simulink model "SF033A_VehSigCdng"  (R2013b)
settings: Solver=FixedStepDiscrete  SolverMode=SingleTasking  StartTime=0.0  StopTime=1  FixedStep=.002  RelTol=1e-3
model workspace (MAT data in the model file):
  SLAMConfig_1_ATPP = [3707764736; 2; 1; 1; 1; 34]
values from neighbouring files (symbols this model uses):
  ARCHGLBPRM_2MILLISEC_SEC_F32 = DataDict.Constant    [SF033A_VehSigCdng_DataDict.m]
  ARCHGLBPRM_PIOVER180_ULS_F32 = DataDict.Constant    [SF033A_VehSigCdng_DataDict.m]
  AUNITCNVN_KPHPERSECPERMTRPERSECSQD_F32 = DataDict.Constant    [SF033A_VehSigCdng_DataDict.m]
  FLTINJ_VEHSIGCDNG_SERLCOMVEHLATA = DataDict.Constant    [SF033A_VehSigCdng_DataDict.m]
  FLTINJ_VEHSIGCDNG_SERLCOMVEHLGTA = DataDict.Constant    [SF033A_VehSigCdng_DataDict.m]
  FLTINJ_VEHSIGCDNG_SERLCOMVEHSPD = DataDict.Constant    [SF033A_VehSigCdng_DataDict.m]
  FLTINJ_VEHSIGCDNG_SERLCOMVEHYAWRATE = DataDict.Constant    [SF033A_VehSigCdng_DataDict.m]
  KPHCONVTOMTRPERSEC_MTRPERSECPERKPH_F32 = DataDict.Constant    [SF033A_VehSigCdng_DataDict.m]
  VehSigCdngDftLatA = DataDict.Calibration    [SF033A_VehSigCdng_DataDict.m]
  VehSigCdngDftLgtA = DataDict.Calibration    [SF033A_VehSigCdng_DataDict.m]
  VehSigCdngDftVehSpd = DataDict.Calibration    [SF033A_VehSigCdng_DataDict.m]
  VehSigCdngDftYawRate = DataDict.Calibration    [SF033A_VehSigCdng_DataDict.m]
  VehSigCdngLatADifThd = DataDict.Calibration    [SF033A_VehSigCdng_DataDict.m]
  VehSigCdngLatASlewRate = DataDict.Calibration    [SF033A_VehSigCdng_DataDict.m]
  VehSigCdngLtgADifThd = DataDict.Calibration    [SF033A_VehSigCdng_DataDict.m]
  VehSigCdngLtgASlewRate = DataDict.Calibration    [SF033A_VehSigCdng_DataDict.m]
  VehSigCdngVehSpdDifThd = DataDict.Calibration    [SF033A_VehSigCdng_DataDict.m]
  VehSigCdngVehSpdSlewRate = DataDict.Calibration    [SF033A_VehSigCdng_DataDict.m]
  VehSigCdngVehYawSlewRate = DataDict.Calibration    [SF033A_VehSigCdng_DataDict.m]
  VehSigCdngYawRateDifThd = DataDict.Calibration    [SF033A_VehSigCdng_DataDict.m]
  VEHSPDOVRDHWTQTHD_HWNWTMTR_F32 = DataDict.Constant    [SF033A_VehSigCdng_DataDict.m]
libraries: NxtrLim x9, CollectionOfReusableBlocks x6, Fil x4, simulink x1
(part 1 of 3)
settings Model: Creator=lzz0tm  LastModifiedBy=bzhf94
settings SolverCC: AutoInsertRateTranBlk=on  InsertRTBMode=Always
settings DataIOCC: LimitDataPoints=off  SaveFormat=Structure  ReturnWorkspaceOutputs=on
settings OptimizationCC: BlockReduction=off  InlineParams=on  ZeroExternalMemoryAtStartup=off  ZeroInternalMemoryAtStartup=off  OptimizeModelRefInitCode=on  LifeSpan=1
settings DebuggingCC: SignalInfNanChecking=error  SignalRangeChecking=warning  UnderspecifiedInitializationDetection=Simplified  SolverPrmCheckMsg=error  InheritedTsInSrcMsg=error  DiscreteInheritContinuousMsg=error  SingleTaskRateTransMsg=error  TasksWithSamePriorityMsg=error  SigSpecEnsureSampleTimeMsg=error  CheckMatrixSingularityMsg=error  ParameterUnderflowMsg=error  ParameterPrecisionLossMsg=error  ParameterTunabilityLossMsg=error  FixptConstUnderflowMsg=warning  FixptConstOverflowMsg=warning  VectorMatrixConversionMsg=error  SignalLabelMismatchMsg=error  UnconnectedInputMsg=error  UnconnectedOutputMsg=error  UnconnectedLineMsg=error  SFcnCompatibilityMsg=error  UniqueDataStoreMsg=warning  BusObjectLabelMismatch=error  RootOutportRequireBusObject=error  AssertControl=DisableAll  ModelReferenceIOMsg=error  ModelReferenceVersionMismatchMessage=warning  ModelReferenceIOMismatchMessage=error  ModelReferenceCSMismatchMessage=warning  ModelReferenceDataLoggingMessage=error  StateNameClashWarn=warning  StrictBusMsg=ErrorOnBusTreatedAsVector  NonBusSignalsTreatedAsBus=error  SFUnexpectedBacktrackingDiag=error  SFInvalidInputDataAccessInChartInitDiag=error  SFNoUnconditionalDefaultTransitionDiag=error  SFTransitionOutsideNaturalParentDiag=error  SFUnconditionalTransitionShadowingDiag=error  SFUndirectedBroadcastEventsDiag=error
settings ModelReferenceCC: ModelReferenceNumInstancesAllowed=Single
settings RTWCC: SystemTargetFile=autosar.tlc  GenCodeOnly=on  TemplateMakefile=ert_default_tmf  Description=AUTOSAR  GenerateReport=on  ProcessScript=autosar_make_rtw_hook  LaunchReport=on
settings CodeAppCC: GenerateComments=off  IgnoreCustomStorageClasses=off  CustomSymbolStrType=$N$R$M  CustomSymbolStrBlkIO=$N$M  SimulinkBlockComments=off
settings STFCustomTargetCC: ParMdlRefBuildCompliant=on  CompOptLevelCompliant=on  IncludeMdlTerminateFcn=off  CombineOutputUpdateFcns=on  SuppressErrorStatus=on  ERTFirstTimeCompliant=on  ERTCustomFileBanners=on  SupportNonFinite=off  SupportComplex=off  SupportContinuousTime=off  SupportNonInlinedSFcns=off  MATLABClassNameForMDSCustomization=Simulink.SoftwareTarget.ERTCustomization  AutosarCompliant=on  GRTInterface=off  SystemTargetFile=autosar.tlc
settings ERTTargetCC: CodeReplacementLibrary=ANSI_C  ConcurrentExecutionCompliant=off  IncludeMdlTerminateFcn=off  SuppressErrorStatus=on  SupportNonFinite=off  SupportComplex=off  ModelStepFunctionPrototypeControlCompliant=off  CPPClassGenCompliant=off  AutosarCompliant=on  InlinedParameterPlacement=NonHierarchical  ERTCustomFileTemplate=example_file_process.tlc  EnableUserReplacementTypes=on

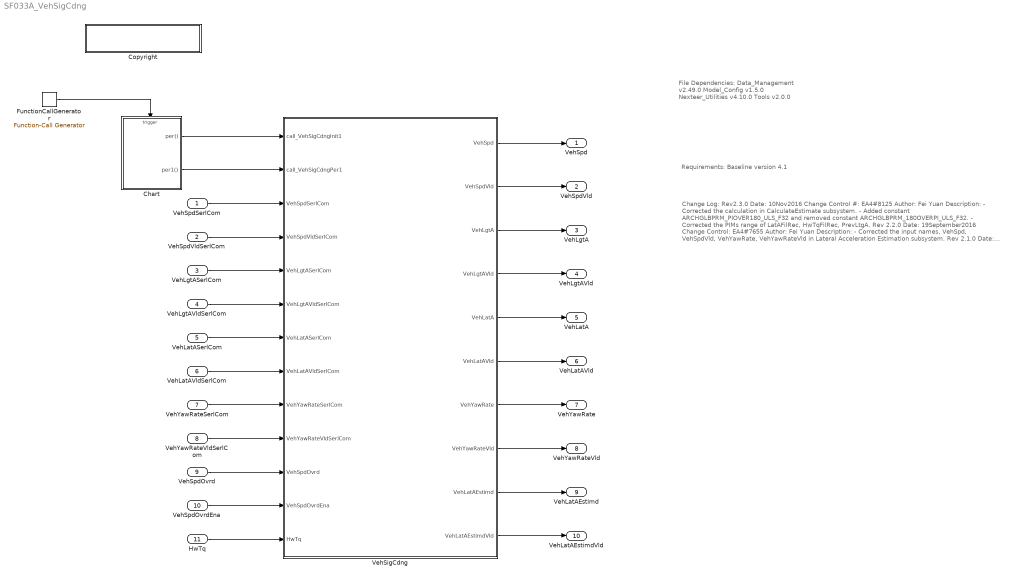
== system SF033A_VehSigCdng ==
  note: File Dependencies:
      |
      | Data_Management v2.49.0
      | Model_Config v1.5.0
      | Nexteer_Utilities v4.10.0
      | Tools v2.0.0
  note: Requirements: Baseline version 4.1
  note: Change Log:
      |
      | Rev2.3.0
      | Date: 10Nov2016
      | Change Control #: EA4#8125
      | Author: Fei Yuan
      | Description:
      | - Corrected the calculation in CalculateEstimate subsystem.
      | - Added constant ARCHGLBPRM_PIOVER180_ULS_F32 and removed constant
      |   ARCHGLBPRM_180OVERPI_ULS_F32.
      | - Corrected the PIMs range of LatAFilRec, HwTqFilRec, PrevLtgA.
      |
      |
      | Rev 2.2.0
      | Date: 19September2016
      | Change Control: EA4#7655
      | Author: Fei Yuan
      | Description:
      | - Corrected the input names, VehSpd, VehSpdVld, VehYawRate, VehYawRateVld in Lateral Acceleration
      | Estimation subsystem.
      |
      |
      | Rev 2.1.0
      | Date: 19August2016
      | Change Control: EA4#6834
      | Author P. Lefler
      | Description:
      | - Update the design so that VehLatAEstimd  is set to VehSpdDdngDftLatA when
      | VehLatAEstimdVld is FALSE and that VehLatAEstimd is calculated from VehSpd and VehYawRate instead of
      | the serial comm messages.
      |
      | - Correct the calculation of VehLatAEstimd. The constants applied to the VehYawRate and
      | VehSpd need to be interchanged.
      |
      |
      | Rev 2.0.0
      | Date: 24May2016
      | Change Control: EA4#3820, EA4#5691
      | Author: P. Lefler
      | Description:
      | EA4#3820 - The calculation and ouput of an estimated Lateral Accleration has been added with an output of validitiy
      | that is determined from the validity of the serial com input signals of Yaw Rate and Vehicle Speed.
      |
      | EA4#5691 - Added inputs and logic to provide override of Vehicle Speed for manufacturing.
      |
      | Rev: 1.1.0
      | Date :16-Oct-2015
      | Change Control #: EA4#2111
      | Author : Sudeep Shankar
      | Description:
      | - Data type of 'VehYawRateVldSerlCom'
      | changed to boolean.
      | - "Data type" of input and output ports changed
      |  to "Inherit: auto" ( Click on a port in the model and
      | select "Signal Attributes")
      |
      |
      | Rev: 1.0.0
      | Date: 26JUN2015
      | Change Control #: EA4#855
      | DRW: Wheatley
      | Description:
      | - Initial EA4 Release, based off
      | 	of EA3 4.0.0 release
  VehSpdSerlCom : Inport  PortDimensions=1
  VehSpdVldSerlCom : Inport  Port=2  PortDimensions=1
  VehLgtASerlCom : Inport  Port=3  PortDimensions=1
  VehLgtAVldSerlCom : Inport  Port=4  PortDimensions=1
  VehLatASerlCom : Inport  Port=5  PortDimensions=1
  VehLatAVldSerlCom : Inport  Port=6  PortDimensions=1
  VehYawRateSerlCom : Inport  Port=7  PortDimensions=1
  VehYawRateVldSerlCom : Inport  Port=8  PortDimensions=1
  VehSpdOvrd : Inport  Port=9  PortDimensions=1
  VehSpdOvrdEna : Inport  Port=10  PortDimensions=1
  HwTq : Inport  Port=11  PortDimensions=1
  Chart : Stateflow chart  TreatAsAtomicUnit=on
  Copyright : Subsystem  Description=|  mask(Copyright Information){none=on}
      | Copyright info block.                                               
      |                                                                     
      | Place copyright information at the top of every subsystem in design.
      mask prompts: none "No parameters"
      mask help: Place copyright information at the top of every subsystem in design.
      mask Display:
      | NxtrConf = 'Nexteer Confidential';
      | 
      | sys = bdroot; %handle for the current model ("system")
      | first = get_param(sys,'Created');
      | first = first(end-3:end);  %year is last four digits
      | 
      | last = get_param(sys,'LastModifiedDate');
      | if isempty(last)
      |     last = datestr(now,'yyyy');
      | else
      |     last = last(end-3:end);
      | end
      | 
      | if strcmp(first,last)
      |     fprintf('%s\nCopyright  %s Nexteer',NxtrConf,first);
      | else
      |     fprintf('%s\n%s%s-%s Nexteer',NxtrConf,char(169),first,last);
      | end
  FunctionCallGenerator : simulink/Ports & Subsystems/Function-Call Generator  sample_time=0.002  numberOfIterations=1
  VehSigCdng : Subsystem
  VehSpd : Outport  PortDimensions=1
  VehSpdVld : Outport  Port=2  PortDimensions=1
  VehLgtA : Outport  Port=3  PortDimensions=1
  VehLgtAVld : Outport  Port=4  PortDimensions=1
  VehLatA : Outport  Port=5  PortDimensions=1
  VehLatAVld : Outport  Port=6  PortDimensions=1
  VehYawRate : Outport  Port=7  PortDimensions=1
  VehYawRateVld : Outport  Port=8  PortDimensions=1
  VehLatAEstimd : Outport  Port=9
  VehLatAEstimdVld : Outport  Port=10
  wires:
  VehLgtASerlCom/1 -> VehSigCdng/5(VehLgtASerlCom)
  VehLgtAVldSerlCom/1 -> VehSigCdng/6(VehLgtAVldSerlCom)
  VehLatASerlCom/1 -> VehSigCdng/7(VehLatASerlCom)
  VehLatAVldSerlCom/1 -> VehSigCdng/8(VehLatAVldSerlCom)
  VehYawRateSerlCom/1 -> VehSigCdng/9(VehYawRateSerlCom)
  VehYawRateVldSerlCom/1 -> VehSigCdng/10(VehYawRateVldSerlCom)
  VehSigCdng/1(VehSpd) -> VehSpd/1
  VehSigCdng/2(VehSpdVld) -> VehSpdVld/1
  VehSigCdng/3(VehLgtA) -> VehLgtA/1
  VehSigCdng/4(VehLgtAVld) -> VehLgtAVld/1
  VehSigCdng/5(VehLatA) -> VehLatA/1
  VehSigCdng/6(VehLatAVld) -> VehLatAVld/1
  VehSigCdng/7(VehYawRate) -> VehYawRate/1
  VehSigCdng/8(VehYawRateVld) -> VehYawRateVld/1
  FunctionCallGenerator/1 -> Chart/Trigger
  Chart/1(per()) -> VehSigCdng/1(call_VehSigCdngInit1)
  Chart/2(per1()) -> VehSigCdng/2(call_VehSigCdngPer1)
  VehSigCdng/9(VehLatAEstimd) -> VehLatAEstimd/1
  VehSigCdng/10(VehLatAEstimdVld) -> VehLatAEstimdVld/1
  VehSpdVldSerlCom/1 -> VehSigCdng/4(VehSpdVldSerlCom)
  VehSpdSerlCom/1 -> VehSigCdng/3(VehSpdSerlCom)
  VehSpdOvrdEna/1 -> VehSigCdng/12(VehSpdOvrdEna)
  HwTq/1 -> VehSigCdng/13(HwTq)
  VehSpdOvrd/1 -> VehSigCdng/11(VehSpdOvrd)

== system SF033A_VehSigCdng/Copyright ==

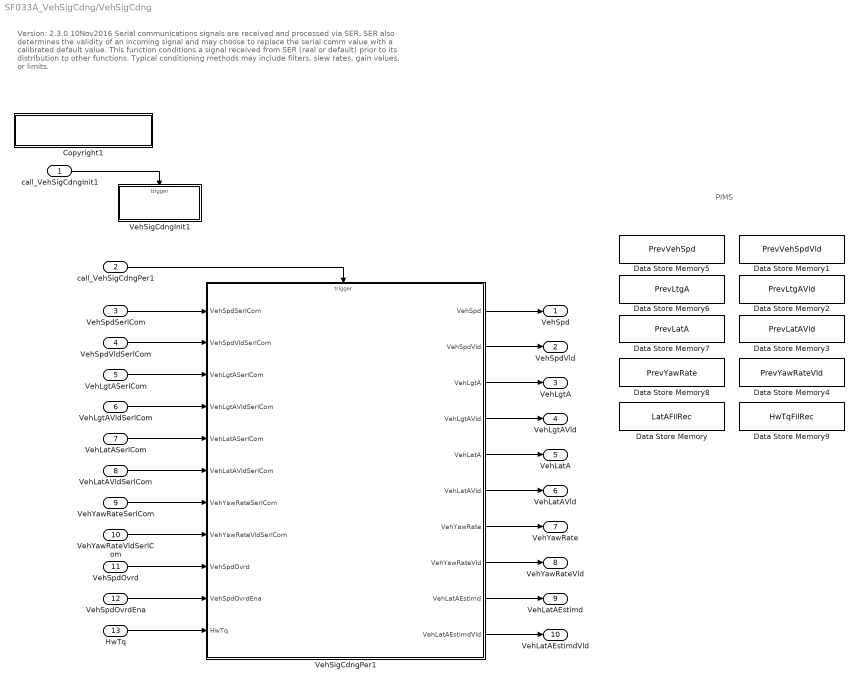
== system SF033A_VehSigCdng/VehSigCdng ==
  note: PIMS
  note: Version:  2.3.0				10Nov2016
      |
      | Serial communications signals are received and processed via SER.  SER also determines the validity of an incoming signal and may choose to replace the serial comm value with a calibrated default value.
      | This function conditions a signal received from SER (real or default) prior to its distribution to other functions.  Typical conditioning methods may include filters, slew rates, gain values, or limits.
  call_VehSigCdngInit1 : Inport
  call_VehSigCdngPer1 : Inport  Port=2
  VehSpdSerlCom : Inport  RequirementInfo="{'linktype_rmi_doors' '00012fc2 (/E-STEER Core/SubSystem Specifications/Application Functions - EA4/SF033A Vehicle Signal Conditioning)' '#SF033A_9' 'true' 'REQ:  SF033A_9' '' } %GIDa_54d4a7a3_9b19_443d_8fc5_eee67838605b"  Port=3  PortDimensions=1
  VehSpdVldSerlCom : Inport  RequirementInfo="{'linktype_rmi_doors' '00012fc2 (/E-STEER Core/SubSystem Specifications/Application Functions - EA4/SF033A Vehicle Signal Conditioning)' '#SF033A_48' 'true' 'REQ:  SF033A_48' '' } %GIDa_072279f1_3b2c_44d1_aaac_d278ed9b7397"  Port=4  PortDimensions=1
  VehLgtASerlCom : Inport  RequirementInfo="{'linktype_rmi_doors' '00012fc2 (/E-STEER Core/SubSystem Specifications/Application Functions - EA4/SF033A Vehicle Signal Conditioning)' '#SF033A_49' 'true' 'REQ:  SF033A_49' '' } %GIDa_26c8abc2_7194_48ce_90af_9aea8ac14bea"  Port=5  PortDimensions=1
  VehLgtAVldSerlCom : Inport  RequirementInfo="{'linktype_rmi_doors' '00012fc2 (/E-STEER Core/SubSystem Specifications/Application Functions - EA4/SF033A Vehicle Signal Conditioning)' '#SF033A_50' 'true' 'REQ:  SF033A_50' '' } %GIDa_37f55aeb_95e9_4e82_a468_aabd9ebeee97"  Port=6  PortDimensions=1
  VehLatASerlCom : Inport  RequirementInfo="{'linktype_rmi_doors' '00012fc2 (/E-STEER Core/SubSystem Specifications/Application Functions - EA4/SF033A Vehicle Signal Conditioning)' '#SF033A_51' 'true' 'REQ:  SF033A_51' '' } %GIDa_d8fc8d11_e171_48fe_b9fc_d65fe4604617"  Port=7  PortDimensions=1
  VehLatAVldSerlCom : Inport  RequirementInfo="{'linktype_rmi_doors' '00012fc2 (/E-STEER Core/SubSystem Specifications/Application Functions - EA4/SF033A Vehicle Signal Conditioning)' '#SF033A_52' 'true' 'REQ:  SF033A_52' '' } %GIDa_d1cab1a5_fbf5_438a_a129_ecd49d66000b"  Port=8  PortDimensions=1
  VehYawRateSerlCom : Inport  RequirementInfo="{'linktype_rmi_doors' '00012fc2 (/E-STEER Core/SubSystem Specifications/Application Functions - EA4/SF033A Vehicle Signal Conditioning)' '#SF033A_53' 'true' 'REQ:  SF033A_53' '' } %GIDa_e3d4cf11_eb0a_4628_8932_e44618244c7f"  Port=9  PortDimensions=1
  VehYawRateVldSerlCom : Inport  RequirementInfo="{'linktype_rmi_doors' '00012fc2 (/E-STEER Core/SubSystem Specifications/Application Functions - EA4/SF033A Vehicle Signal Conditioning)' '#SF033A_54' 'true' 'REQ:  SF033A_54' '' } %GIDa_0d1894a8_7423_4afc_9a9d_b2e7187f4361"  Port=10  PortDimensions=1
  VehSpdOvrd : Inport  RequirementInfo="{'linktype_rmi_doors' '00012fc2 (/E-STEER Core/SubSystem Specifications/Application Functions - EA4/SF033A Vehicle Signal Conditioning)' '#SF033A_55' 'true' 'REQ:  SF033A_55' '' } %GIDa_6a43a7d4_88db_4c6f_8f53_b974adffb088"  Port=11  PortDimensions=1
  VehSpdOvrdEna : Inport  RequirementInfo="{'linktype_rmi_doors' '00012fc2 (/E-STEER Core/SubSystem Specifications/Application Functions - EA4/SF033A Vehicle Signal Conditioning)' '#SF033A_56' 'true' 'REQ:  SF033A_56' '' } %GIDa_18bae755_d713_41e5_97b7_5a248150ee5f"  Port=12  PortDimensions=1
  HwTq : Inport  RequirementInfo="{'linktype_rmi_doors' '00012fc2 (/E-STEER Core/SubSystem Specifications/Application Functions - EA4/SF033A Vehicle Signal Conditioning)' '#SF033A_57' 'true' 'REQ:  SF033A_57' '' } %GIDa_76451758_dfda_400b_b021_5024d294a7ba"  Port=13  PortDimensions=1
  Copyright1 : Subsystem  Description=|  mask(Copyright Information){none=on}
      | Copyright info block.                                               
      |                                                                     
      | Place copyright information at the top of every subsystem in design.
      mask prompts: none "No parameters"
      mask help: Place copyright information at the top of every subsystem in design.
      mask Display:
      | NxtrConf = 'Nexteer Confidential';
      | 
      | sys = bdroot; %handle for the current model ("system")
      | first = get_param(sys,'Created');
      | first = first(end-3:end);  %year is last four digits
      | 
      | last = get_param(sys,'LastModifiedDate');
      | if isempty(last)
      |     last = datestr(now,'yyyy');
      | else
      |     last = last(end-3:end);
      | end
      | 
      | if strcmp(first,last)
      |     fprintf('%s\nCopyright  %s Nexteer',NxtrConf,first);
      | else
      |     fprintf('%s\n%s%s-%s Nexteer',NxtrConf,char(169),first,last);
      | end
  Data Store Memory : DataStoreMemory  RequirementInfo="{'linktype_rmi_doors' '00012fc2 (/E-STEER Core/SubSystem Specifications/Application Functions - EA4/SF033A Vehicle Signal Conditioning)' '#SF033A_95' 'true' 'REQ:  SF033A_95' '' } %GIDa_0c5846ab_92bd_4d29_8a45_462a927c3a81"  DataStoreName=LatAFilRec  InitialValue=struct('FilSt',single(0),'FilGain',single(0))  OutDataTypeStr=Bus: FilLpRec1  StateMustResolveToSignalObject=on
  Data Store Memory1 : DataStoreMemory  DataStoreName=PrevVehSpdVld  StateMustResolveToSignalObject=on
  Data Store Memory2 : DataStoreMemory  DataStoreName=PrevLtgAVld  StateMustResolveToSignalObject=on
  Data Store Memory3 : DataStoreMemory  DataStoreName=PrevLatAVld  StateMustResolveToSignalObject=on
  Data Store Memory4 : DataStoreMemory  DataStoreName=PrevYawRateVld  StateMustResolveToSignalObject=on
  Data Store Memory5 : DataStoreMemory  DataStoreName=PrevVehSpd  StateMustResolveToSignalObject=on
  Data Store Memory6 : DataStoreMemory  DataStoreName=PrevLtgA  StateMustResolveToSignalObject=on
  Data Store Memory7 : DataStoreMemory  DataStoreName=PrevLatA  StateMustResolveToSignalObject=on
  Data Store Memory8 : DataStoreMemory  DataStoreName=PrevYawRate  StateMustResolveToSignalObject=on
  Data Store Memory9 : DataStoreMemory  RequirementInfo="{'linktype_rmi_doors' '00012fc2 (/E-STEER Core/SubSystem Specifications/Application Functions - EA4/SF033A Vehicle Signal Conditioning)' '#SF033A_70' 'true' 'REQ:  SF033A_70' '' ; 'linktype_rmi_doors' '00012fc2 (/E-STEER Core/SubSystem Specifications/Application Functions - EA4/SF033A Vehicle Signal Conditioning)' '#SF033A_106' 'true' 'REQ:  SF033A_106' '' } %GIDa_2e2802be_6404_4db6_874c_aabd103a4acc"  DataStoreName=HwTqFilRec  InitialValue=[]  StateMustResolveToSignalObject=on
  VehSigCdngInit1 : Subsystem  TreatAsAtomicUnit=on
  VehSigCdngPer1 : Subsystem
  VehSpd : Outport  RequirementInfo="{'linktype_rmi_doors' '00012fc2 (/E-STEER Core/SubSystem Specifications/Application Functions - EA4/SF033A Vehicle Signal Conditioning)' '#SF033A_11' 'true' 'REQ:  SF033A_11' '' } %GIDa_233b96dc_1a76_410d_9511_57228fcb2a2c"  PortDimensions=1
  VehSpdVld : Outport  RequirementInfo="{'linktype_rmi_doors' '00012fc2 (/E-STEER Core/SubSystem Specifications/Application Functions - EA4/SF033A Vehicle Signal Conditioning)' '#SF033A_58' 'true' 'REQ:  SF033A_58' '' } %GIDa_ac8eeb31_52c9_4a8f_b3bc_984b37742cf2"  Port=2  PortDimensions=1
  VehLgtA : Outport  RequirementInfo="{'linktype_rmi_doors' '00012fc2 (/E-STEER Core/SubSystem Specifications/Application Functions - EA4/SF033A Vehicle Signal Conditioning)' '#SF033A_59' 'true' 'REQ:  SF033A_59' '' } %GIDa_690e0b41_3963_43a6_9a31_eb7586529f9d"  Port=3  PortDimensions=1
  VehLgtAVld : Outport  RequirementInfo="{'linktype_rmi_doors' '00012fc2 (/E-STEER Core/SubSystem Specifications/Application Functions - EA4/SF033A Vehicle Signal Conditioning)' '#SF033A_61' 'true' 'REQ:  SF033A_61' '' } %GIDa_d05753c6_a2a8_4d16_8807_9f672ca9e552"  Port=4  PortDimensions=1
  VehLatA : Outport  RequirementInfo="{'linktype_rmi_doors' '00012fc2 (/E-STEER Core/SubSystem Specifications/Application Functions - EA4/SF033A Vehicle Signal Conditioning)' '#SF033A_62' 'true' 'REQ:  SF033A_62' '' } %GIDa_87d4c65b_0136_48cb_a577_93593ee03691"  Port=5  PortDimensions=1
  VehLatAVld : Outport  RequirementInfo="{'linktype_rmi_doors' '00012fc2 (/E-STEER Core/SubSystem Specifications/Application Functions - EA4/SF033A Vehicle Signal Conditioning)' '#SF033A_65' 'true' 'REQ:  SF033A_65' '' } %GIDa_16cef6e8_4176_4268_935b_383d23a79d5c"  Port=6  PortDimensions=1
  VehYawRate : Outport  RequirementInfo="{'linktype_rmi_doors' '00012fc2 (/E-STEER Core/SubSystem Specifications/Application Functions - EA4/SF033A Vehicle Signal Conditioning)' '#SF033A_63' 'true' 'REQ:  SF033A_63' '' } %GIDa_5922fcb3_f223_4d4a_a6ba_bb2ffcc33926"  Port=7  PortDimensions=1
  VehYawRateVld : Outport  RequirementInfo="{'linktype_rmi_doors' '00012fc2 (/E-STEER Core/SubSystem Specifications/Application Functions - EA4/SF033A Vehicle Signal Conditioning)' '#SF033A_64' 'true' 'REQ:  SF033A_64' '' } %GIDa_ede16489_acab_444a_8f38_7e62a6621c77"  Port=8  PortDimensions=1
  VehLatAEstimd : Outport  RequirementInfo="{'linktype_rmi_doors' '00012fc2 (/E-STEER Core/SubSystem Specifications/Application Functions - EA4/SF033A Vehicle Signal Conditioning)' '#SF033A_60' 'true' 'REQ:  SF033A_60' '' } %GIDa_bd1c9d75_d3fa_4d5a_9ec3_8a13a125d70d"  Port=9
  VehLatAEstimdVld : Outport  RequirementInfo="{'linktype_rmi_doors' '00012fc2 (/E-STEER Core/SubSystem Specifications/Application Functions - EA4/SF033A Vehicle Signal Conditioning)' '#SF033A_66' 'true' 'REQ:  SF033A_66' '' } %GIDa_e77b9470_d33a_498a_a2de_20107a9a1a32"  Port=10
  wires:
  VehLgtASerlCom/1 -> VehSigCdngPer1/3(VehLgtASerlCom)
  VehSpdSerlCom/1 -> VehSigCdngPer1/1(VehSpdSerlCom)
  call_VehSigCdngPer1/1 -> VehSigCdngPer1/Trigger
  VehSpdVldSerlCom/1 -> VehSigCdngPer1/2(VehSpdVldSerlCom)
  VehLatASerlCom/1 -> VehSigCdngPer1/5(VehLatASerlCom)
  call_VehSigCdngInit1/1 -> VehSigCdngInit1/Trigger
  VehLgtAVldSerlCom/1 -> VehSigCdngPer1/4(VehLgtAVldSerlCom)
  VehLatAVldSerlCom/1 -> VehSigCdngPer1/6(VehLatAVldSerlCom)
  VehYawRateSerlCom/1 -> VehSigCdngPer1/7(VehYawRateSerlCom)
  VehYawRateVldSerlCom/1 -> VehSigCdngPer1/8(VehYawRateVldSerlCom)
  VehSigCdngPer1/1(VehSpd) -> VehSpd/1
  VehSigCdngPer1/2(VehSpdVld) -> VehSpdVld/1
  VehSigCdngPer1/3(VehLgtA) -> VehLgtA/1
  VehSigCdngPer1/5(VehLatA) -> VehLatA/1
  VehSigCdngPer1/4(VehLgtAVld) -> VehLgtAVld/1
  VehSigCdngPer1/6(VehLatAVld) -> VehLatAVld/1
  VehSigCdngPer1/7(VehYawRate) -> VehYawRate/1
  VehSigCdngPer1/8(VehYawRateVld) -> VehYawRateVld/1
  VehSigCdngPer1/9(VehLatAEstimd) -> VehLatAEstimd/1
  VehSigCdngPer1/10(VehLatAEstimdVld) -> VehLatAEstimdVld/1
  VehSpdOvrd/1 -> VehSigCdngPer1/9(VehSpdOvrd)
  VehSpdOvrdEna/1 -> VehSigCdngPer1/10(VehSpdOvrdEna)
  HwTq/1 -> VehSigCdngPer1/11(HwTq)

== system SF033A_VehSigCdng/VehSigCdng/Copyright1 ==

== system SF033A_VehSigCdng/VehSigCdng/VehSigCdngInit1 ==
  function : TriggerPort  TriggerType=function-call
  CopyRight2 : Subsystem  Description=|  mask(Copyright Information){none=on}
      | Copyright info block.                                               
      |                                                                     
      | Place copyright information at the top of every subsystem in design.
      mask prompts: none "No parameters"
      mask help: Place copyright information at the top of every subsystem in design.
      mask Display:
      | NxtrConf = 'Nexteer Confidential';
      | 
      | sys = bdroot; %handle for the current model ("system")
      | first = get_param(sys,'Created');
      | first = first(end-3:end);  %year is last four digits
      | 
      | last = get_param(sys,'LastModifiedDate');
      | if isempty(last)
      |     last = datestr(now,'yyyy');
      | else
      |     last = last(end-3:end);
      | end
      | 
      | if strcmp(first,last)
      |     fprintf('%s -- Copyright %s Nexteer',NxtrConf,first)
      | else
      |     fprintf('%s -- %s%s- %s Nexteer',NxtrConf,char(169),first,last)
      | end
  FilLpInit : Fil/FilLpInit  RequirementInfo="{'linktype_rmi_doors' '00012fc2 (/E-STEER Core/SubSystem Specifications/Application Functions - EA4/SF033A Vehicle Signal Conditioning)' '#SF033A_95' 'true' 'REQ:  SF033A_95' '' } %GIDa_7accb8cc_27e6_4227_a4fe_4cab8debe218"  Ic=0  Ts=ARCHGLBPRM_2MILLISEC_SEC_F32  Freq=VehSigCdngLatAFilFrq  StVar=LatAFilRec
  FilLpInit1 : Fil/FilLpInit  RequirementInfo="{'linktype_rmi_doors' '00012fc2 (/E-STEER Core/SubSystem Specifications/Application Functions - EA4/SF033A Vehicle Signal Conditioning)' '#SF033A_70' 'true' 'REQ:  SF033A_70' '' ; 'linktype_rmi_doors' '00012fc2 (/E-STEER Core/SubSystem Specifications/Application Functions - EA4/SF033A Vehicle Signal Conditioning)' '#SF033A_106' 'true' 'REQ:  SF033A_106' '' } %GIDa_a1695ab3_73dc_4f0d_88aa_6746bdcfefc1"  Ic=0  Ts=ARCHGLBPRM_2MILLISEC_SEC_F32  Freq=single(0.1)  StVar=HwTqFilRec

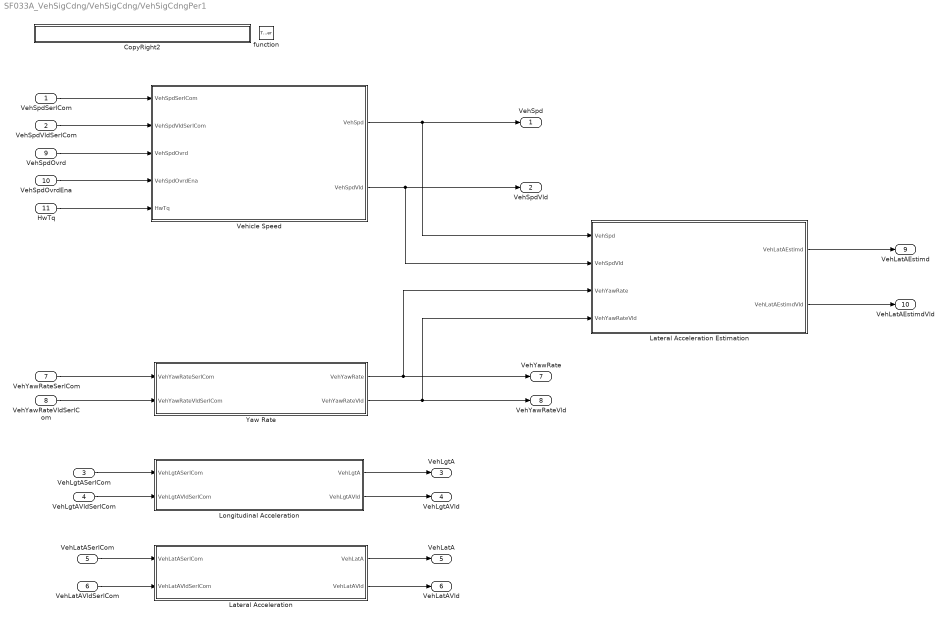
== system SF033A_VehSigCdng/VehSigCdng/VehSigCdngPer1 ==
  VehSpdSerlCom : Inport  PortDimensions=1
  VehSpdVldSerlCom : Inport  Port=2  PortDimensions=1
  VehLgtASerlCom : Inport  Port=3  PortDimensions=1
  VehLgtAVldSerlCom : Inport  Port=4  PortDimensions=1
  VehLatASerlCom : Inport  Port=5  PortDimensions=1
  VehLatAVldSerlCom : Inport  Port=6  PortDimensions=1
  VehYawRateSerlCom : Inport  Port=7  PortDimensions=1
  VehYawRateVldSerlCom : Inport  Port=8  PortDimensions=1
  VehSpdOvrd : Inport  Port=9  PortDimensions=1
  VehSpdOvrdEna : Inport  Port=10  PortDimensions=1
  HwTq : Inport  Port=11  PortDimensions=1
  function : TriggerPort  TriggerType=function-call  PortDimensions=1
  CopyRight2 : Subsystem  Description=|  mask(Copyright Information){none=on}
      | Copyright info block.                                               
      |                                                                     
      | Place copyright information at the top of every subsystem in design.
      mask prompts: none "No parameters"
      mask help: Place copyright information at the top of every subsystem in design.
      mask Display:
      | NxtrConf = 'Nexteer Confidential';
      | 
      | sys = bdroot; %handle for the current model ("system")
      | first = get_param(sys,'Created');
      | first = first(end-3:end);  %year is last four digits
      | 
      | last = get_param(sys,'LastModifiedDate');
      | if isempty(last)
      |     last = datestr(now,'yyyy');
      | else
      |     last = last(end-3:end);
      | end
      | 
      | if strcmp(first,last)
      |     fprintf('%s -- Copyright %s Nexteer',NxtrConf,first)
      | else
      |     fprintf('%s -- %s%s- %s Nexteer',NxtrConf,char(169),first,last)
      | end
  Lateral Acceleration : Subsystem
  Lateral Acceleration Estimation : Subsystem
  Longitudinal Acceleration : Subsystem
  Vehicle Speed : Subsystem
  "Yaw Rate " : Subsystem
  VehSpd : Outport  PortDimensions=1
  VehSpdVld : Outport  Port=2  PortDimensions=1
  VehLgtA : Outport  Port=3  PortDimensions=1
  VehLgtAVld : Outport  Port=4  PortDimensions=1
  VehLatA : Outport  Port=5  PortDimensions=1
  VehLatAVld : Outport  Port=6  PortDimensions=1
  VehYawRate : Outport  Port=7  PortDimensions=1
  VehYawRateVld : Outport  Port=8  PortDimensions=1
  VehLatAEstimd : Outport  Port=9
  VehLatAEstimdVld : Outport  Port=10
  wires:
  Vehicle Speed/1(VehSpd) -> VehSpd/1, Lateral Acceleration Estimation/1(VehSpd)
  Vehicle Speed/2(VehSpdVld) -> VehSpdVld/1, Lateral Acceleration Estimation/2(VehSpdVld)
  VehLgtASerlCom/1 -> Longitudinal Acceleration/1(VehLgtASerlCom)
  VehLgtAVldSerlCom/1 -> Longitudinal Acceleration/2(VehLgtAVldSerlCom)
  Longitudinal Acceleration/1(VehLgtA) -> VehLgtA/1
  Longitudinal Acceleration/2(VehLgtAVld) -> VehLgtAVld/1
  VehLatASerlCom/1 -> Lateral Acceleration/1(VehLatASerlCom)
  VehLatAVldSerlCom/1 -> Lateral Acceleration/2(VehLatAVldSerlCom)
  Lateral Acceleration/1(VehLatA) -> VehLatA/1
  Lateral Acceleration/2(VehLatAVld) -> VehLatAVld/1
  "Yaw Rate "/1(VehYawRate) -> Lateral Acceleration Estimation/3(VehYawRate), VehYawRate/1
  "Yaw Rate "/2(VehYawRateVld) -> Lateral Acceleration Estimation/4(VehYawRateVld), VehYawRateVld/1
  Lateral Acceleration Estimation/2(VehLatAEstimdVld) -> VehLatAEstimdVld/1
  Lateral Acceleration Estimation/1(VehLatAEstimd) -> VehLatAEstimd/1
  VehSpdSerlCom/1 -> Vehicle Speed/1(VehSpdSerlCom)
  VehYawRateSerlCom/1 -> "Yaw Rate "/1(VehYawRateSerlCom)
  VehSpdVldSerlCom/1 -> Vehicle Speed/2(VehSpdVldSerlCom)
  VehYawRateVldSerlCom/1 -> "Yaw Rate "/2(VehYawRateVldSerlCom)
  VehSpdOvrd/1 -> Vehicle Speed/3(VehSpdOvrd)
  VehSpdOvrdEna/1 -> Vehicle Speed/4(VehSpdOvrdEna)
  HwTq/1 -> Vehicle Speed/5(HwTq)

== system SF033A_VehSigCdng/VehSigCdng/VehSigCdngInit1/CopyRight2 ==

== system SF033A_VehSigCdng/VehSigCdng/VehSigCdngPer1/CopyRight2 ==

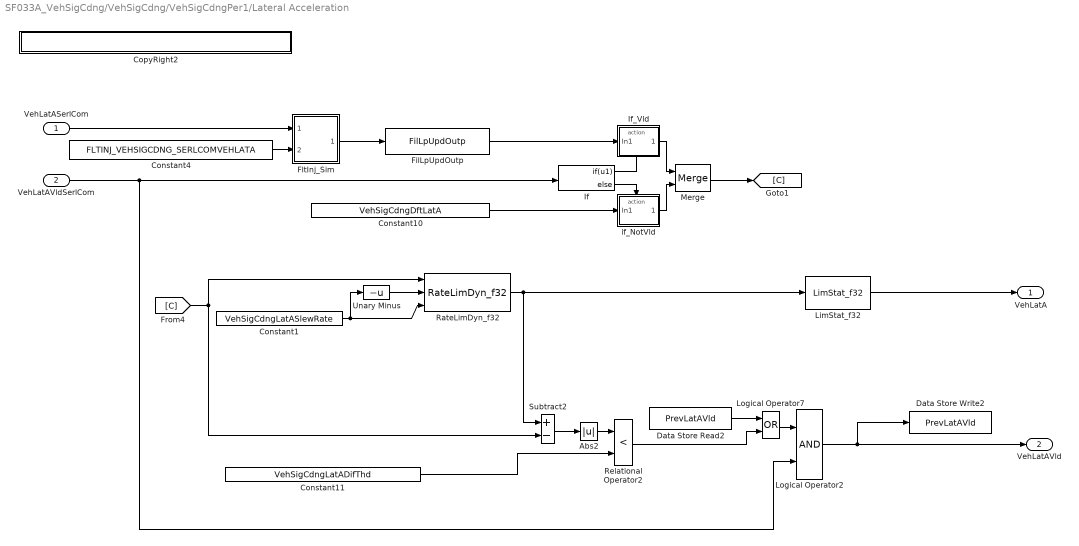
== system SF033A_VehSigCdng/VehSigCdng/VehSigCdngPer1/Lateral Acceleration ==
  VehLatASerlCom : Inport  RequirementInfo="{'linktype_rmi_doors' '00012fc2 (/E-STEER Core/SubSystem Specifications/Application Functions - EA4/SF033A Vehicle Signal Conditioning)' '#SF033A_95' 'true' 'REQ:  SF033A_95' '' ; 'linktype_rmi_doors' '00012fc2 (/E-STEER Core/SubSystem Specifications/Application Functions - EA4/SF033A Vehicle Signal Conditioning)' '#SF033A_96' 'true' 'REQ:  SF033A_96' '' } %GIDa_c753c921_7e04_496c_95fa_487e63ca1125"  PortDimensions=1
  VehLatAVldSerlCom : Inport  RequirementInfo="{'linktype_rmi_doors' '00012fc2 (/E-STEER Core/SubSystem Specifications/Application Functions - EA4/SF033A Vehicle Signal Conditioning)' '#SF033A_95' 'true' 'REQ:  SF033A_95' '' ; 'linktype_rmi_doors' '00012fc2 (/E-STEER Core/SubSystem Specifications/Application Functions - EA4/SF033A Vehicle Signal Conditioning)' '#SF033A_96' 'true' 'REQ:  SF033A_96' '' } %GIDa_b07f8488_028f_4994_885b_452029bb587c"  Port=2  PortDimensions=1
  Abs2 : Abs  RequirementInfo="{'linktype_rmi_doors' '00012fc2 (/E-STEER Core/SubSystem Specifications/Application Functions - EA4/SF033A Vehicle Signal Conditioning)' '#SF033A_94' 'true' 'REQ:  SF033A_94' '' } %GIDa_5a62b5de_cc32_48b8_924f_7873d67ebb50"
  Constant1 : Constant  RequirementInfo="{'linktype_rmi_doors' '00012fc2 (/E-STEER Core/SubSystem Specifications/Application Functions - EA4/SF033A Vehicle Signal Conditioning)' '#SF033A_92' 'true' 'REQ:  SF033A_92' '' } %GIDa_eb3c9be8_1e78_47b8_835b_b4d0d1ae4ea5"  Value=VehSigCdngLatASlewRate
  Constant10 : Constant  RequirementInfo="{'linktype_rmi_doors' '00012fc2 (/E-STEER Core/SubSystem Specifications/Application Functions - EA4/SF033A Vehicle Signal Conditioning)' '#SF033A_96' 'true' 'REQ:  SF033A_96' '' } %GIDa_91ae6bfc_aa5f_43f0_9820_b24db602beb2"  Value=VehSigCdngDftLatA
  Constant11 : Constant  RequirementInfo="{'linktype_rmi_doors' '00012fc2 (/E-STEER Core/SubSystem Specifications/Application Functions - EA4/SF033A Vehicle Signal Conditioning)' '#SF033A_94' 'true' 'REQ:  SF033A_94' '' } %GIDa_a0d1b654_bbde_4064_8b63_104446a06a98"  Value=VehSigCdngLatADifThd
  Constant4 : Constant  RequirementInfo="{'linktype_rmi_doors' '00012fc2 (/E-STEER Core/SubSystem Specifications/Application Functions - EA4/SF033A Vehicle Signal Conditioning)' '#SF033A_109' 'true' 'REQ:  SF033A_109' '' } %GIDa_1542dcc9_2bda_4046_a838_588fdf05564c"  Value=FLTINJ_VEHSIGCDNG_SERLCOMVEHLATA
  CopyRight2 : Subsystem  Description=|  mask(Copyright Information){none=on}
      | Copyright info block.                                               
      |                                                                     
      | Place copyright information at the top of every subsystem in design.
      mask prompts: none "No parameters"
      mask help: Place copyright information at the top of every subsystem in design.
      mask Display:
      | NxtrConf = 'Nexteer Confidential';
      | 
      | sys = bdroot; %handle for the current model ("system")
      | first = get_param(sys,'Created');
      | first = first(end-3:end);  %year is last four digits
      | 
      | last = get_param(sys,'LastModifiedDate');
      | if isempty(last)
      |     last = datestr(now,'yyyy');
      | else
      |     last = last(end-3:end);
      | end
      | 
      | if strcmp(first,last)
      |     fprintf('%s -- Copyright %s Nexteer',NxtrConf,first)
      | else
      |     fprintf('%s -- %s%s- %s Nexteer',NxtrConf,char(169),first,last)
      | end
  Data Store Read2 : DataStoreRead  DataStoreName=PrevLatAVld
  Data Store Write2 : DataStoreWrite  DataStoreName=PrevLatAVld
  FilLpUpdOutp : Fil/FilLpUpdOutp  RequirementInfo="{'linktype_rmi_doors' '00012fc2 (/E-STEER Core/SubSystem Specifications/Application Functions - EA4/SF033A Vehicle Signal Conditioning)' '#SF033A_95' 'true' 'REQ:  SF033A_95' '' } %GIDa_7953da50_dcec_437e_8f3a_a91fadd74616"  StVar=LatAFilRec
      settings: AttributesFormatString=StVar: %<StVar>
  FltInj_Sim : Subsystem  RequirementInfo="{'linktype_rmi_doors' '00012fc2 (/E-STEER Core/SubSystem Specifications/Application Functions - EA4/SF033A Vehicle Signal Conditioning)' '#SF033A_109' 'true' 'REQ:  SF033A_109' '' } %GIDa_932a3e69_52ef_4461_8f18_f05710d5a38c"  TreatAsAtomicUnit=on  VariantControl=FltInj_sim
  If : If  RequirementInfo="{'linktype_rmi_doors' '00012fc2 (/E-STEER Core/SubSystem Specifications/Application Functions - EA4/SF033A Vehicle Signal Conditioning)' '#SF033A_95' 'true' 'REQ:  SF033A_95' '' } %GIDa_c0a6e30e_f7f2_4ae2_8bd5_78b2454898f8"  IfExpression=u1
  If_Vld : Subsystem  RequirementInfo="{'linktype_rmi_doors' '00012fc2 (/E-STEER Core/SubSystem Specifications/Application Functions - EA4/SF033A Vehicle Signal Conditioning)' '#SF033A_95' 'true' 'REQ:  SF033A_95' '' } %GIDa_1a18b11a_c2c8_4315_9c86_e615b348a758"  TreatAsAtomicUnit=on
  LimStat_f32 : NxtrLim/LimStat_f32  RequirementInfo="{'linktype_rmi_doors' '00012fc2 (/E-STEER Core/SubSystem Specifications/Application Functions - EA4/SF033A Vehicle Signal Conditioning)' '#SF033A_68' 'true' 'REQ:  SF033A_68' '' } %GIDa_565a3834_33b0_48c8_bda9_39c0135f306e"  LoLim=VEHLATAMINLIM_MTRPERSECSQD_F32  HiLim=VEHLATAMAXLIM_MTRPERSECSQD_F32
      settings: AttributesFormatString=|
      | Low Limit: %<LoLim>
      | High Limit:%<HiLim>
  Logical Operator2 : Logic  RequirementInfo="{'linktype_rmi_doors' '00012fc2 (/E-STEER Core/SubSystem Specifications/Application Functions - EA4/SF033A Vehicle Signal Conditioning)' '#SF033A_94' 'true' 'REQ:  SF033A_94' '' } %GIDa_b93f9bf8_8c8d_49ea_9a19_9c3aa95c8c46"  AllPortsSameDT=off  OutDataTypeStr=boolean
  Logical Operator7 : Logic  RequirementInfo={} %GIDa_0d11762d_d5f3_4b81_9adb_b6696da2d055  Operator=OR  AllPortsSameDT=off  OutDataTypeStr=boolean
  Merge : Merge  RequirementInfo="{'linktype_rmi_doors' '00012fc2 (/E-STEER Core/SubSystem Specifications/Application Functions - EA4/SF033A Vehicle Signal Conditioning)' '#SF033A_95' 'true' 'REQ:  SF033A_95' '' ; 'linktype_rmi_doors' '00012fc2 (/E-STEER Core/SubSystem Specifications/Application Functions - EA4/SF033A Vehicle Signal Conditioning)' '#SF033A_96' 'true' 'REQ:  SF033A_96' '' } %GIDa_50b13ee9_892c_4d3d_bbe5_336da9314504"
  RateLimDyn_f32 : NxtrLim/RateLimDyn_f32  RequirementInfo="{'linktype_rmi_doors' '00012fc2 (/E-STEER Core/SubSystem Specifications/Application Functions - EA4/SF033A Vehicle Signal Conditioning)' '#SF033A_92' 'true' 'REQ:  SF033A_92' '' ; 'linktype_rmi_doors' '00012fc2 (/E-STEER Core/SubSystem Specifications/Application Functions - EA4/SF033A Vehicle Signal Conditioning)' '#SF033A_94' 'true' 'REQ:  SF033A_94' '' } %GIDa_0d31863d_131a_49d1_8cc1_c6725db574da"  StVar=PrevLatA  Ts=ARCHGLBPRM_2MILLISEC_SEC_F32
      settings: AttributesFormatString=StVar: %<StVar>
  Relational Operator2 : RelationalOperator  RequirementInfo="{'linktype_rmi_doors' '00012fc2 (/E-STEER Core/SubSystem Specifications/Application Functions - EA4/SF033A Vehicle Signal Conditioning)' '#SF033A_94' 'true' 'REQ:  SF033A_94' '' } %GIDa_3326bf16_8950_4b24_9351_d042ae9d2a16"  Operator=<  OutDataTypeStr=boolean
  Subtract2 : Sum  RequirementInfo="{'linktype_rmi_doors' '00012fc2 (/E-STEER Core/SubSystem Specifications/Application Functions - EA4/SF033A Vehicle Signal Conditioning)' '#SF033A_94' 'true' 'REQ:  SF033A_94' '' } %GIDa_65766f24_b4bf_467f_8826_b376a6accbe4"  Inputs=+-
  Unary Minus : UnaryMinus  RequirementInfo="{'linktype_rmi_doors' '00012fc2 (/E-STEER Core/SubSystem Specifications/Application Functions - EA4/SF033A Vehicle Signal Conditioning)' '#SF033A_92' 'true' 'REQ:  SF033A_92' '' } %GIDa_9db1bcd7_2dd4_4c44_abbf_6f46c37a848d"
  if_NotVld : Subsystem  RequirementInfo="{'linktype_rmi_doors' '00012fc2 (/E-STEER Core/SubSystem Specifications/Application Functions - EA4/SF033A Vehicle Signal Conditioning)' '#SF033A_96' 'true' 'REQ:  SF033A_96' '' } %GIDa_7c77875e_bce5_4868_a3fd_3acfe9def7a2"  TreatAsAtomicUnit=on
  VehLatA : Outport  RequirementInfo="{'linktype_rmi_doors' '00012fc2 (/E-STEER Core/SubSystem Specifications/Application Functions - EA4/SF033A Vehicle Signal Conditioning)' '#SF033A_95' 'true' 'REQ:  SF033A_95' '' ; 'linktype_rmi_doors' '00012fc2 (/E-STEER Core/SubSystem Specifications/Application Functions - EA4/SF033A Vehicle Signal Conditioning)' '#SF033A_96' 'true' 'REQ:  SF033A_96' '' } %GIDa_7f59c02f_ea69_49d8_a568_b23d8c83c3ac"  PortDimensions=1
  VehLatAVld : Outport  RequirementInfo="{'linktype_rmi_doors' '00012fc2 (/E-STEER Core/SubSystem Specifications/Application Functions - EA4/SF033A Vehicle Signal Conditioning)' '#SF033A_95' 'true' 'REQ:  SF033A_95' '' ; 'linktype_rmi_doors' '00012fc2 (/E-STEER Core/SubSystem Specifications/Application Functions - EA4/SF033A Vehicle Signal Conditioning)' '#SF033A_96' 'true' 'REQ:  SF033A_96' '' } %GIDa_788d65cc_2879_46cd_a78a_510659937fc3"  Port=2  PortDimensions=1
  wires:
  Constant4/1 -> FltInj_Sim/2(Enum)
  VehLatASerlCom/1 -> FltInj_Sim/1(Signal)
  Subtract2/1 -> Abs2/1
  Abs2/1 -> Relational Operator2/1
  Constant11/1 -> Relational Operator2/2
  Relational Operator2/1 -> Logical Operator7/2
  VehLatAVldSerlCom/1 -> Logical Operator2/2, If/1
  [C] -> RateLimDyn_f32/1, Subtract2/2
  LimStat_f32/1 -> VehLatA/1
  FltInj_Sim/1(Out1) -> FilLpUpdOutp/1
  Data Store Read2/1 -> Logical Operator7/1
  Logical Operator7/1 -> Logical Operator2/1
  Logical Operator2/1 -> VehLatAVld/1, Data Store Write2/1
  Constant1/1 -> Unary Minus/1, RateLimDyn_f32/3
  If/1 -> If_Vld/Action
  If/2 -> if_NotVld/Action
  If_Vld/1(Out1) -> Merge/1
  if_NotVld/1(Out1) -> Merge/2
  Constant10/1 -> if_NotVld/1(In1)
  FilLpUpdOutp/1 -> If_Vld/1(In1)
  Merge/1 -> [C]
  RateLimDyn_f32/1 -> LimStat_f32/1, Subtract2/1
  Unary Minus/1 -> RateLimDyn_f32/2

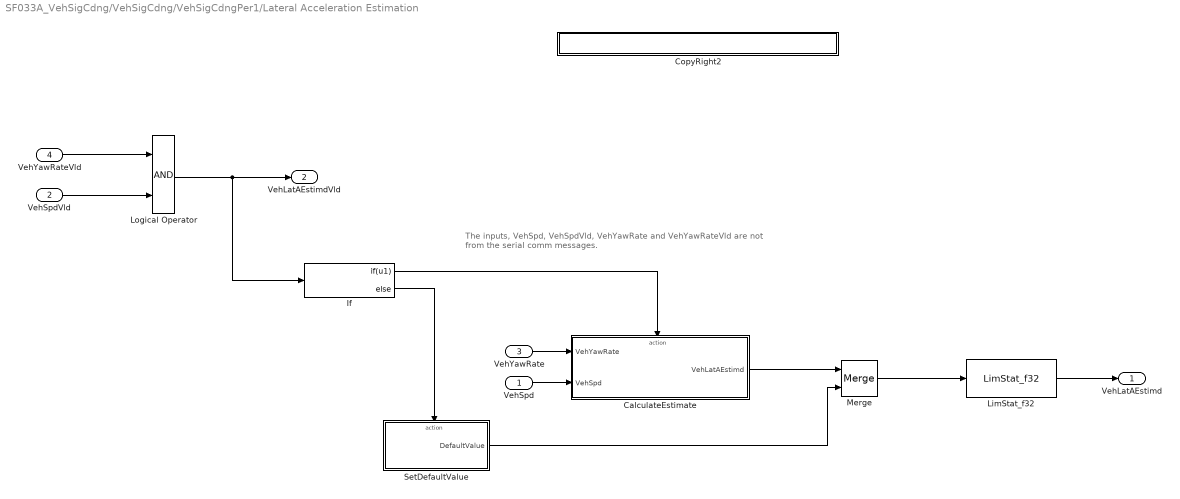
== system SF033A_VehSigCdng/VehSigCdng/VehSigCdngPer1/Lateral Acceleration Estimation ==
  note: The inputs, VehSpd, VehSpdVld, VehYawRate and VehYawRateVld are
      | not from the serial comm messages.
  VehSpd : Inport  RequirementInfo="{'linktype_rmi_doors' '00012fc2 (/E-STEER Core/SubSystem Specifications/Application Functions - EA4/SF033A Vehicle Signal Conditioning)' '#SF033A_97' 'true' 'REQ:  SF033A_97' '' } %GIDa_f8e53e87_7948_4f08_9377_76b53feb2acb"  PortDimensions=1
  VehSpdVld : Inport  RequirementInfo="{'linktype_rmi_doors' '00012fc2 (/E-STEER Core/SubSystem Specifications/Application Functions - EA4/SF033A Vehicle Signal Conditioning)' '#SF033A_98' 'true' 'REQ:  SF033A_98' '' } %GIDa_9b7da564_7d8c_4b40_a8e4_43123ce5b0e7"  Port=2  PortDimensions=1
  VehYawRate : Inport  RequirementInfo="{'linktype_rmi_doors' '00012fc2 (/E-STEER Core/SubSystem Specifications/Application Functions - EA4/SF033A Vehicle Signal Conditioning)' '#SF033A_97' 'true' 'REQ:  SF033A_97' '' } %GIDa_761e70fd_018d_4686_bbe1_e2c2c028d829"  Port=3  PortDimensions=1
  VehYawRateVld : Inport  RequirementInfo="{'linktype_rmi_doors' '00012fc2 (/E-STEER Core/SubSystem Specifications/Application Functions - EA4/SF033A Vehicle Signal Conditioning)' '#SF033A_98' 'true' 'REQ:  SF033A_98' '' } %GIDa_1f43f7b4_8419_48de_bec9_b5f0c6554f08"  Port=4  PortDimensions=1
  CalculateEstimate : Subsystem  RequirementInfo="{'linktype_rmi_doors' '00012fc2 (/E-STEER Core/SubSystem Specifications/Application Functions - EA4/SF033A Vehicle Signal Conditioning)' '#SF033A_97' 'true' 'REQ:  SF033A_97' '' } %GIDa_196caa3f_9c94_490c_a64d_ca74cf09c24c"  TreatAsAtomicUnit=on
  CopyRight2 : Subsystem  Description=|  mask(Copyright Information){none=on}
      | Copyright info block.                                               
      |                                                                     
      | Place copyright information at the top of every subsystem in design.
      mask prompts: none "No parameters"
      mask help: Place copyright information at the top of every subsystem in design.
      mask Display:
      | NxtrConf = 'Nexteer Confidential';
      | 
      | sys = bdroot; %handle for the current model ("system")
      | first = get_param(sys,'Created');
      | first = first(end-3:end);  %year is last four digits
      | 
      | last = get_param(sys,'LastModifiedDate');
      | if isempty(last)
      |     last = datestr(now,'yyyy');
      | else
      |     last = last(end-3:end);
      | end
      | 
      | if strcmp(first,last)
      |     fprintf('%s -- Copyright %s Nexteer',NxtrConf,first)
      | else
      |     fprintf('%s -- %s%s- %s Nexteer',NxtrConf,char(169),first,last)
      | end
  If : If  RequirementInfo="{'linktype_rmi_doors' '00012fc2 (/E-STEER Core/SubSystem Specifications/Application Functions - EA4/SF033A Vehicle Signal Conditioning)' '#SF033A_97' 'true' 'REQ:  SF033A_97' '' ; 'linktype_rmi_doors' '00012fc2 (/E-STEER Core/SubSystem Specifications/Application Functions - EA4/SF033A Vehicle Signal Conditioning)' '#SF033A_99' 'true' 'REQ:  SF033A_99' '' } %GIDa_6f9353c9_236b_4606_b454_bfcf76696e21"  IfExpression=u1
  LimStat_f32 : NxtrLim/LimStat_f32  RequirementInfo="{'linktype_rmi_doors' '00012fc2 (/E-STEER Core/SubSystem Specifications/Application Functions - EA4/SF033A Vehicle Signal Conditioning)' '#SF033A_68' 'true' 'REQ:  SF033A_68' '' } %GIDa_b2ed47c8_c2cd_4dfd_8946_5fc14991f1aa"  LoLim=LATACCEESTIMDMINLIM_MTRPERSECSQD_F32  HiLim=LATACCEESTIMDMAXLIM_MTRPERSECSQD_F32
      settings: AttributesFormatString=|
      | Low Limit: %<LoLim>
      | High Limit:%<HiLim>
  Logical Operator : Logic  RequirementInfo="{'linktype_rmi_doors' '00012fc2 (/E-STEER Core/SubSystem Specifications/Application Functions - EA4/SF033A Vehicle Signal Conditioning)' '#SF033A_98' 'true' 'REQ:  SF033A_98' '' } %GIDa_4573f6d7_0a17_4c9d_94fc_15d04dcd9c9e"  AllPortsSameDT=off  OutDataTypeStr=boolean
  Merge : Merge  RequirementInfo="{'linktype_rmi_doors' '00012fc2 (/E-STEER Core/SubSystem Specifications/Application Functions - EA4/SF033A Vehicle Signal Conditioning)' '#SF033A_97' 'true' 'REQ:  SF033A_97' '' ; 'linktype_rmi_doors' '00012fc2 (/E-STEER Core/SubSystem Specifications/Application Functions - EA4/SF033A Vehicle Signal Conditioning)' '#SF033A_99' 'true' 'REQ:  SF033A_99' '' } %GIDa_8b591c39_5c12_49c8_8873_6e8cc9df527f"
  SetDefaultValue : Subsystem  RequirementInfo="{'linktype_rmi_doors' '00012fc2 (/E-STEER Core/SubSystem Specifications/Application Functions - EA4/SF033A Vehicle Signal Conditioning)' '#SF033A_99' 'true' 'REQ:  SF033A_99' '' } %GIDa_10b47bab_4ee0_4325_93d1_2e25d317a1a3"  TreatAsAtomicUnit=on
  VehLatAEstimd : Outport  RequirementInfo="{'linktype_rmi_doors' '00012fc2 (/E-STEER Core/SubSystem Specifications/Application Functions - EA4/SF033A Vehicle Signal Conditioning)' '#SF033A_97' 'true' 'REQ:  SF033A_97' '' ; 'linktype_rmi_doors' '00012fc2 (/E-STEER Core/SubSystem Specifications/Application Functions - EA4/SF033A Vehicle Signal Conditioning)' '#SF033A_99' 'true' 'REQ:  SF033A_99' '' } %GIDa_59a5dedb_3562_4b86_b5d4_afed65b2e988"
  VehLatAEstimdVld : Outport  RequirementInfo="{'linktype_rmi_doors' '00012fc2 (/E-STEER Core/SubSystem Specifications/Application Functions - EA4/SF033A Vehicle Signal Conditioning)' '#SF033A_98' 'true' 'REQ:  SF033A_98' '' } %GIDa_606b77ad_d6f8_42ce_a01a_c9320a6edb9f"  Port=2
  wires:
  VehSpdVld/1 -> Logical Operator/2
  VehYawRateVld/1 -> Logical Operator/1
  Logical Operator/1 -> If/1, VehLatAEstimdVld/1
  LimStat_f32/1 -> VehLatAEstimd/1
  If/1 -> CalculateEstimate/Action
  If/2 -> SetDefaultValue/Action
  CalculateEstimate/1(VehLatAEstimd) -> Merge/1
  SetDefaultValue/1(DefaultValue) -> Merge/2
  VehYawRate/1 -> CalculateEstimate/1(VehYawRate)
  VehSpd/1 -> CalculateEstimate/2(VehSpd)
  Merge/1 -> LimStat_f32/1
